simulink model "untitled1"  (R2024b)
settings: Solver=VariableStepAuto  StartTime=0.0  StopTime=70000  RelTol=1e-3
values from neighbouring files (symbols this model uses):
  r = 50.65    [modele_siplifie.m]
  tau1 = 30    [modele_siplifie.m]
settings Model: Creator=medam  LastModifiedBy=medam

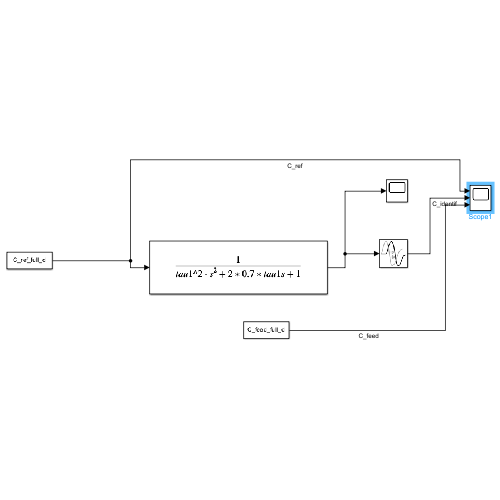
[thumbnail: Simulink's stored preview of the top-level diagram]
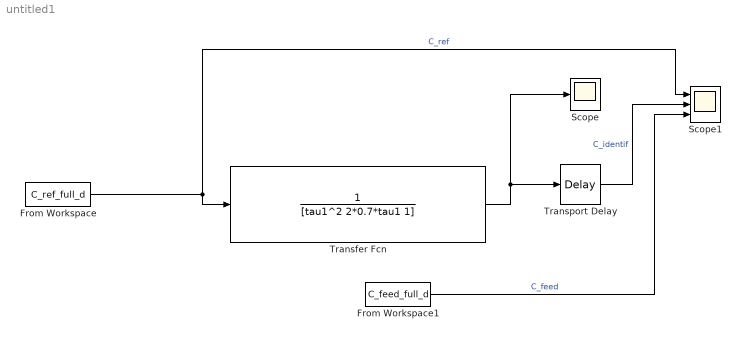
== system untitled1 ==
  From Workspace : FromWorkspace  VariableName=C_ref_full_d
  From Workspace1 : FromWorkspace  VariableName=C_feed_full_d
  Scope : Scope
  Scope1 : Scope  NumInputPorts=3
  Transfer Fcn : TransferFcn  Denominator=[tau1^2 2*0.7*tau1 1]
  Transport Delay : TransportDelay  DelayTime=r
  wires:
  Transfer Fcn/1 -> Transport Delay/1, Scope/1
  Transport Delay/1 -> Scope1/2  "C_identif"
  From Workspace1/1 -> Scope1/3  "C_feed"
  From Workspace/1 -> Scope1/1, Transfer Fcn/1  "C_ref"
